simulink model "project_model (1)"  (R2025a)
settings: Solver=FixedStepAuto  StartTime=0.0  StopTime=10.0  FixedStep=1e-3  RelTol=1e-3  EnableMultiTasking=on
undefined symbols (not defined in the file): D2, PTB9
libraries: frdmk64flib x3, etargetslib x2
settings Model: ExtModeTrigDuration=5  Creator=justi  LastModifiedBy=justi
settings OptimizationCC: DefaultParameterBehavior=Inlined  EnhancedBackFolding=on  PassReuseOutputArgsAs=Individual arguments  ZeroExternalMemoryAtStartup=off  ZeroInternalMemoryAtStartup=off  MaxStackSize=64  OptimizeBlockOrder=speed  DifferentSizesBufferReuse=on  OptimizationCustomize=off  EfficientTunableParamExpr=on
settings DebuggingCC: ParameterTunabilityLossMsg=error
settings HardwareCC: ProdBitPerPointer=32.0  ProdBitPerSizeT=32.0  ProdBitPerPtrDiffT=32.0  ProdLargestAtomicInteger=Long  ProdLargestAtomicFloat=Double  ProdWordSize=32.0  ProdHWDeviceType=ARM Compatible->ARM Cortex
settings SFSimCC: MATLABDynamicMemAlloc=off
settings RTWCC: SystemTargetFile=ert.tlc  HardwareBoard=NXP FRDM-K64F  TLCOptions="-aInlineSetEventsForThisBaseRateFcn=TLC_FALSE -aSuppressMultiTaskScheduler=TLC_FALSE  -aRateBasedStepFcn=0"  TemplateMakefile=ert_default_tmf  Toolchain=GNU Tools for ARM Embedded Processors  Description=Embedded Coder
settings CodeAppCC: ForceParamTrailComments=on  IgnoreCustomStorageClasses=off  OperatorAnnotations=on  SimulinkDataObjDesc=on  SFDataObjDesc=on  InsertBlockDesc=on
settings ERTTargetCC: ExtModeTransport=4.0  ExtModeStaticAlloc=off  ExtModeMexFile=sendToCommService  ExtModeIntrfLevel=Level1

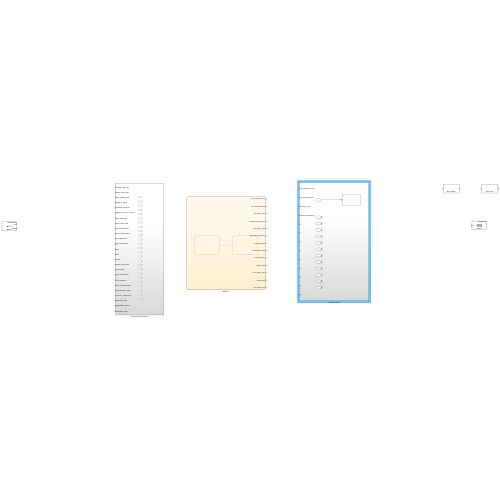
[thumbnail: Simulink's stored preview of the top-level diagram]
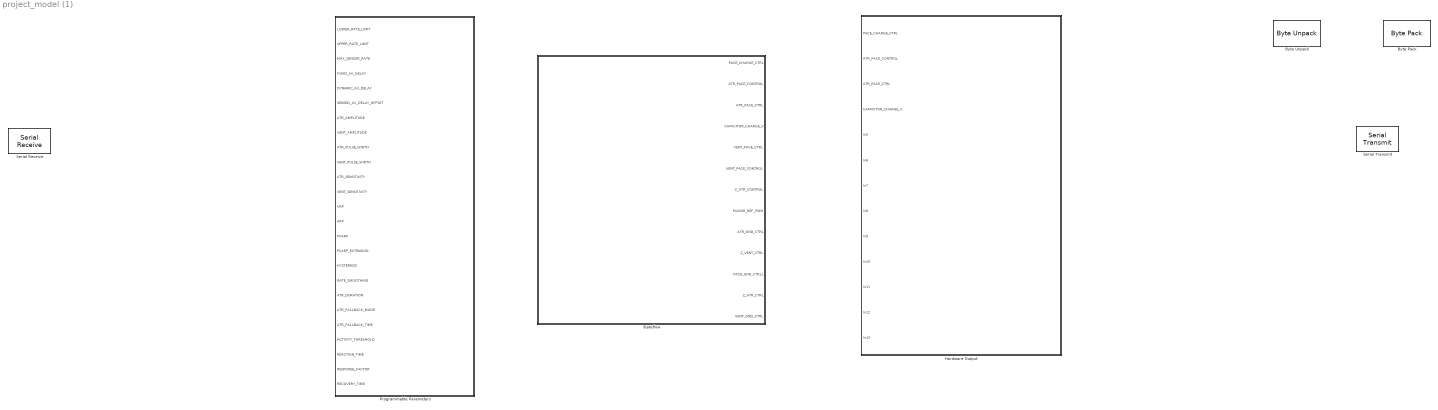
== system project_model (1) ==
  Byte Pack : etargetslib/Byte Pack  datatypes={'single'}  byteAlign=1
  Byte Unpack : etargetslib/Byte Unpack  dimensions={[1]}  datatypes={'single'}  byteAlign=1
      settings: LibrarySourceBlock=embeddedtargetslib/Host Communication/Byte Unpack
  Hardware Output : Subsystem
  Programmable Parameters : Subsystem
  Serial Receive : frdmk64flib/Serial Receive  SCIModule=0  Baudrate=uint32(9600)  Parity=None  StopBits=1  HardwareFlowControl=None  ByteOrder=LittleEndian  DataType=uint8  DataLength=10  BlockingMode=off  OutputStatus=on  SampleTime=-1
  Serial Transmit : frdmk64flib/Serial Transmit  SCIModule=0  Baudrate=uint32(9600)  Parity=None  StopBits=1  HardwareFlowControl=None  ByteOrder=LittleEndian  BlockingMode=on  OutputStatus=off
  "Stateflow " : Stateflow chart  TreatAsAtomicUnit=on

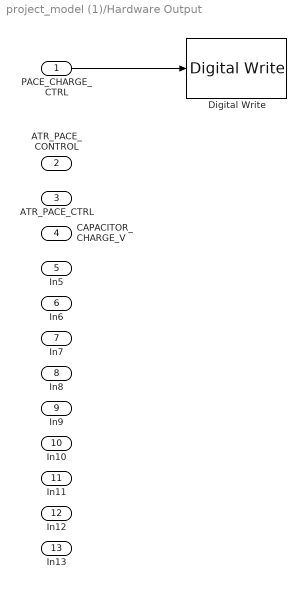
== system project_model (1)/Hardware Output ==
  PACE_CHARGE_CTRL : Inport
  ATR_PACE_CONTROL : Inport  Port=2
  ATR_PACE_CTRL : Inport  Port=3
  CAPACITOR_CHARGE_V : Inport  Port=4
  In5 : Inport  Port=5
  In6 : Inport  Port=6
  In7 : Inport  Port=7
  In8 : Inport  Port=8
  In9 : Inport  Port=9
  In10 : Inport  Port=10
  In11 : Inport  Port=11
  In12 : Inport  Port=12
  In13 : Inport  Port=13
  Digital Write : frdmk64flib/Digital Write  Whichpin=PTB9 (D2)
  wires:
  PACE_CHARGE_CTRL/1 -> Digital Write/1

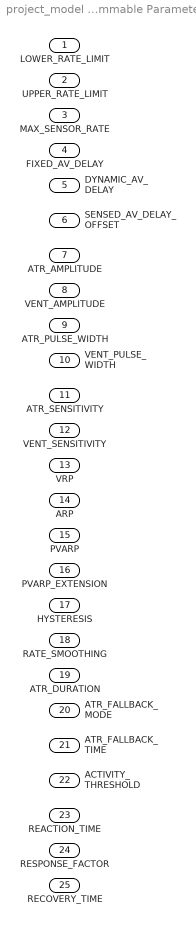
== system project_model (1)/Programmable Parameters ==
  LOWER_RATE_LIMIT : Inport
  UPPER_RATE_LIMIT : Inport  Port=2
  MAX_SENSOR_RATE : Inport  Port=3
  FIXED_AV_DELAY : Inport  Port=4
  DYNAMIC_AV_DELAY : Inport  Port=5
  SENSED_AV_DELAY_OFFSET : Inport  Port=6
  ATR_AMPLITUDE : Inport  Port=7
  VENT_AMPLITUDE : Inport  Port=8
  ATR_PULSE_WIDTH : Inport  Port=9
  VENT_PULSE_WIDTH : Inport  Port=10
  ATR_SENSITIVITY : Inport  Port=11
  VENT_SENSITIVITY : Inport  Port=12
  VRP : Inport  Port=13
  ARP : Inport  Port=14
  PVARP : Inport  Port=15
  PVARP_EXTENSION : Inport  Port=16
  HYSTERESIS : Inport  Port=17
  RATE_SMOOTHING : Inport  Port=18
  ATR_DURATION : Inport  Port=19
  ATR_FALLBACK_MODE : Inport  Port=20
  ATR_FALLBACK_TIME : Inport  Port=21
  ACTIVITY_THRESHOLD : Inport  Port=22
  REACTION_TIME : Inport  Port=23
  RESPONSE_FACTOR : Inport  Port=24
  RECOVERY_TIME : Inport  Port=25

== stateflow chart project_model (1)/Stateflow  ==
  state Discharge
    PACE_CHARGE_CTRL=0;
    PACE_GND_CTRL=1;
    ATR_PACE_CTRL=0;
    ATR_GND_CTRL=0;
    Z_ATR_CTRL=0;
    Z_VENT_CTRL=0;
    VENT_GND_CTRL=0;
    VENT_PACE_CTRL=0;
  state Charge
    ATR_PACE_CTRL=0;
    VENT_PACE_CTRL=0;
    PACING_REF_PWM=2000;%todo
    CAPACITOR_CHARGE_V=5;
    PACE_CHARGE_CTRL=1;
  (default) -> Charge
  Charge -> Discharge : [after(0.54,sec)]
  Discharge -> Charge : [after(0.54,sec)]
  data: PACE_CHARGE_CTRL output; ATR_PACE_CONTROL output; ATR_PACE_CTRL output; CAPACITOR_CHARGE_V output; VENT_PACE_CTRL output; VENT_PACE_CONTROL output; Z_ATR_CONTROL output; PACING_REF_PWM output; ATR_GND_CTRL output; Z_VENT_CTRL output; PACE_GND_CTRLL output; Z_ATR_CTRL output; VENT_GND_CTRL output
